simulink model "vehicle_hostmodel_2022b_RoadrunnerFinal"  (R2022b)
settings: Solver=VariableStepAuto  StartTime=0.0  StopTime=inf  RelTol=1e-3
model workspace (MAT data in the model file):
  finalint = 0
  firstWarning = 1
  originalScenarioChecksum = '114339432DE22364D47BB28FC96DC10C'
undefined symbols (not defined in the file): Acceleration, ActorID, AngularVelocity, curvature, DefaultGear, DEND_B, DEND_S, DEND_T, direction, DiscIntNeverNeededParam, driving, gradbp, L, LF, LR, matlabshared, MAX_BRAKE, MAX_STEER, MAX_TORQUE, MCAR, MIN_BRAKE, MIN_STEER, MIN_TORQUE, NUMD_B, NUMD_S, NUMD_T, Pitch, Position, psi_o, R, Roll, RRdamp, SceneInfo, session, sigbuilder_block, STEER_RATIO, stopSign_ID, Tdead, thetaRefs, TL_ID, TrackWidth, Ts, ts, Vdead, Velocity, WB, X_o, xRef2s, Y_o, Yaw, yRef2, yRef2s
libraries: simulink x10, drivingscenarioandsensors x8, slrealtimeutilitieslib x7, slrealtimeiplib x7, simulink_extras x4, drivingvehiclecontroller x3, robotalgslib x2, slpidlib x2, trackingutilitieslib x2, eeGeneralControl x1, mpcadaslib x1, drivinglib x1
(part 4 of 4)

== matlab function vehicle_hostmodel_2022b_RoadrunnerFinal/Function-Call Subsystem/MATLAB Function2 ==
  data: EgoPosition input; MIOPos input; curvature input; MIOVel input; V_i input; xd output; yd output; laneL input; laneR input; V_desired input; LCinProgress output
function [xd,yd,LCinProgress] = traj(EgoPosition,MIOPos,curvature,MIOVel, V_i, laneL, laneR, V_desired)
Vx_i =0;Vx_f=0;Vy_i=0;Vy_f=0;Ax_i=0;Ax_f=0;Ay_i=0;Ay_f=0;T_i=0;T_f=0;V_f=0;A_f=0;x_set=0;y_set=0;theta4=0;

P = zeros(6,6);
% xq = zeros(1,size(RefPath,1)); yq = zeros(1,size(RefPath,2));
EgoPosition(1,2)=-EgoPosition(1,2)
x_init= EgoPosition(1,1)+5; y_init = EgoPosition(1,2);
% xq = RefPath(:,1)'; 
% yq = RefPath(:,2)';
num_foc_t = 98;
V_max= V_desired; ad_n=0; vd_n=MIOVel; wd_n=vd_n*curvature;
lane_width = 3.6 * (laneL-laneR); % +1 if left of current lane and -1 if right of current lane
xd = zeros(num_foc_t+1,1); 
yd = zeros(num_foc_t+1,1);
xf =0; 
yf = 0;

    %xf = [EgoPosition(1,1)+ MIOPos(1) ]; yf = [ EgoPosition(1,2)+ MIOPos(2) + lane_width];  
    xf = [EgoPosition(1,1)+ 40 ]; yf = [ EgoPosition(1,2)+ 1.2*lane_width]; % 80
    V_f = V_max;
    W_f = V_f*curvature;
    A_f = 0;

    %dist2crash = sqrt((x_init-MIOPos(1))^2+(y_init-MIOPos(2))^2);
    %dist2crash = 40;
    %T_f = abs(dist2crash/(MIOVel-V_i));
    T_f = 3;
    P = [1, T_i, T_i^2, T_i^3, T_i^4, T_i^5;
         0, 1, 2*T_i, 3*T_i^2, 4*T_i^3, 5*T_i^4;
         0, 0, 2, 6*T_i, 12*T_i^2, 20*T_i^3;
         1, T_f, T_f^2, T_f^3, T_f^4, T_f^5;
         0, 1, 2*T_f, 3*T_f^2, 4*T_f^3, 5*T_f^4;
         0, 0, 2, 6*T_f, 12*T_f^2, 20*T_f^3];

%     mtang4 = (yq(1,index+2)-yq(1,index+1))/(xq(1,index+2)-xq(1,index+1));

    Vx_i = vd_n*cos(theta4); 
    Vy_i = vd_n*sin(theta4); 
    Ax_i = ad_n*cos(theta4)-vd_n*sin(theta4)*wd_n; 
    Ay_i = ad_n*sin(theta4)+vd_n*cos(theta4)*wd_n;

%     if(xq(index+2)-xq(index+1)<0)
%         theta_4 = pi + atan(mtang4);
%     else
%         theta_4 = atan(mtang4);
%     end

    theta_4 =0;
    Vx_f = V_f*cos(theta_4); % curvature angle
    Vy_f = V_f*sin(theta_4);
    Ax_f = A_f*cos(theta_4)-V_f*sin(theta_4)*W_f;
    Ay_f = A_f*sin(theta_4)+V_f*cos(theta_4)*W_f;

    g1 = [x_init; Vx_i; Ax_i; xf; Vx_f; Ax_f];
    g2 = [y_init; Vy_i; Ay_i; yf; Vy_f; Ay_f];

    a_coeff = P\g1;
    b_coeff = P\g2;
    
    td = T_i;
    scatter(x_init,y_init,'go')
    hold on; 
    scatter(xf,yf,'ro')
    hold on;
    
    for f = 1:(num_foc_t+1)
        xd(f,1) = [1,td,td^2,td^3,td^4,td^5]*a_coeff 
        yd(f,1) = [1,td,td^2,td^3,td^4,td^5]*b_coeff
        td = td + (T_f - T_i)/num_foc_t;
        scatter(xd(f,1),yd(f,1),'y.');
    end

LCinProgress = 1;

% hold on;
end

== matlab function vehicle_hostmodel_2022b_RoadrunnerFinal/Controllers/Subsystem3/Subsystem2/MATLAB Function ==
  data: u input; accel output; decel output
function [accel, decel] = fcn(u)
if(u>0)
    accel=u; decel=0;
elseif(u<0)
    accel=0; decel=-u;
else
    accel=0;decel=0;
end

== matlab function vehicle_hostmodel_2022b_RoadrunnerFinal/Controllers/MATLAB Function2 ==
  data: v input; RefVelCmd output; curvature input
function RefVelCmd = fcn(v,curvature)

    if abs(curvature) >= 0 && abs(curvature) <= 1e-2
        RefVelCmd = v;
    else
        r = 1/abs(curvature);
        RefVelCmd = min(v,sqrt(9.81*r*.2));
    end

== matlab function vehicle_hostmodel_2022b_RoadrunnerFinal/Vehicle Dynamics/Info2ActorState/MATLAB Function1 ==
  data: Xdot input; Velocity output; Ydot input; Zdot input
function Velocity = fcn(Xdot, Ydot, Zdot)

Velocity = [Xdot Ydot, Zdot];

== matlab function vehicle_hostmodel_2022b_RoadrunnerFinal/MATLAB Function ==
  data: ttc output; dist output; left output; right output; LL_avail output; RL_avail output; tend2stay output; ego input; act input; LaneBounds input; RoadSpeed input; ego_vel output; stay output; LL_Change output; RL_Change output; y_lane output; LCinProgress input
 function [ttc,dist,left,right,LL_avail,RL_avail,tend2stay,ego_vel,stay,LL_Change,RL_Change,y_lane] = fcn(ego,act,LaneBounds,RoadSpeed, LCinProgress)                       


%% Major tasks to look into

% Check the performance while transitioning into another lane 
% Lane change output when the ego on extreme lanes.
% Develop code to handle lane changes on road curvatures
% Integrate with the trajectory generation and check the perfomance 
% Convert the code to ego vehicle coordinates


%%
%define some parameters
r_c = 20; %range considered to MIOs
t_min =  2;

num_actors = length(act.Actors);
%num_lanes = length(LaneBounds.LaneBoundaries)-1;


%% Using sensor data 
% TracksNum = Tracking.NumTracks;
% 
% 
% for t = 1:TracksNum
%     ObjectID(t) = Tracking.Tracks(t).ObjectClassID;
%     TrackPos(:,t) = Tracking.Tracks(t).State(1:2:5);
%     TrackVel(:,t) = Tracking.Tracks(t).State(2:2:6);

%% ego position and  velocity magnitude
ego_pos = ego.Position;
ego_vel = ego.Velocity(1);  % velocity

%ttc: (array) : agent.relative position / abs(relative velocity)
ttc = zeros(1,num_actors);
left = zeros(1,num_actors);
right = zeros(1,num_actors);

dist =  zeros(1,num_actors);
tend2stay=1;

%%
y_lane = zeros(1,length(LaneBounds.LaneBoundaries))

for l=1:length(y_lane)
    y_lane(l)=LaneBounds.LaneBoundaries(l).Coordinates(end,2)
end

%%
for i= 1:num_actors

    % Grab actor positions and velocities
    actor_pos = act.Actors(i).Position;   
    actor_vel = act.Actors(i).Velocity(1);  % x-component velocity

    %relative velocity of the agent
    rel_vel = actor_vel - ego_vel;


    %% Check if the actor is within a r_c range. If it is out of range, pass lane change as '1' automatically.

   dist(i) = norm([actor_pos(1) actor_pos(2)]-[ego_pos(1) ego_pos(2)]);
        
    if dist(i) > r_c
        left(i)=1;
        right(i)=1;
        continue
    end

    %% Check if the actor is in the same lane as that of ego

    % If the actor and ego are in the same lane, it is considered a lead/following vehicle in the same lane and by defualt, the lane change flag is 1.

    if (actor_pos(2)< (ego_pos(2)+0.5) && actor_pos(2) > (ego_pos(2)-0.5))
        if (rel_vel < 0 && ego_vel < (RoadSpeed+5) && actor_pos(1) > ego_pos(1) )
            left(i) =1;
            right(i)=1;
            tend2stay=0;        % we need to incorporate too slow condition even when the relative velocity is greater than 0.

        elseif (rel_vel < 0 && ego_vel < (RoadSpeed+5) && actor_pos(1) < ego_pos(1) )
            left(i) =1;
            right(i)=1;
            tend2stay=1;
        end

        continue
    end

    
    %% calculate ttc for the rest of the vehicles


    ttc(i) = (actor_pos(1)-ego_pos(1))/abs(rel_vel);

    % checking conditions for other surrounding actors

    % all actors on the left lane of the ego vehicle
%%
    if actor_pos(2)-ego_pos(2) > 0  

        if and(rel_vel>0, ttc(i) > t_min)  % target vehicles on the front of ego vehicle (any lane)
    
            left(i)=1; 
            right(i)=1;
    
        elseif (ttc(i)<0 && rel_vel<0 && abs(ttc(i)) > t_min)    % target vehicle on the back of ego vehicle (ttc<0) (any lane)
            left(i) =1;
            right(i)=1;
    
        else 
            left(i) =0;
            right(i)=1;
    
        end

    % all actors on the right lane of the ego vehicle

    elseif actor_pos(2)-ego_pos(2) < 0
         
        if and(rel_vel>0, ttc(i) > t_min)  % target vehicles on the front of ego vehicle (any lane)
    
            left(i)=1;
            right(i)=1;
    
        elseif (ttc(i)<0 && rel_vel<0 && abs(ttc(i)) > t_min)    % target vehicle on the back of ego vehicle (ttc<0) (any lane)
            left(i) =1;
            right(i)=1;
    
        else 
            left(i) =1;
            right(i)=0;
    
        end
    end
%%

end

%% check if the vehicle is in the extreme end lanes

    if ego_pos(2)<y_lane(1) && ego_pos(2)>y_lane(2)

        LL=0; RL=1;
    elseif ego_pos(2) > y_lane(end) && ego_pos(2) < y_lane(end-1)
        RL=0; LL=1;
    else 

        RL=1;LL=1;
    end

%%
LL_avail = all(left) %&& LL;

RL_avail = all(right) %&& RL               %&& ~lcLeft ; this can be decided later 


%% final commands

stay = tend2stay || ~(tend2stay || LL_avail || RL_avail);
LL_Change =  ~tend2stay && LL_avail ;

RL_Change =  ~tend2stay && RL_avail && ~LL_Change ;
LCFlag = ~stay;
if LCFlag && LCinProgress
    LCFlag = false;
    stay = ~LCFlag;
end

%% 






end

== matlab function vehicle_hostmodel_2022b_RoadrunnerFinal/Vehicle Dynamics/Info2ActorState/MATLAB Function2 ==
  data: aX input; Acceleration output; aY input; aZ input
function Acceleration = fcn(aX, aY, aZ)

Acceleration = [aX aY, aZ];

== matlab function vehicle_hostmodel_2022b_RoadrunnerFinal/Vehicle Dynamics/Info2ActorState/MATLAB Function3 ==
  data: phiDot input; AngularVelocity output; thetaDot input; psiDot input
function AngularVelocity = fcn(phiDot, thetaDot, psiDot)

AngularVelocity = [phiDot thetaDot, psiDot];

== stateflow chart vehicle_hostmodel_2022b_RoadrunnerFinal/Vehicle Dynamics/VehicleDynamics/engine-steer-brake dynamics/GearSelection1 ==
  state Park
    CurrGear = 0;
  state Reverse
    CurrGear = -1;
  state drive
    CurrGear = 1;
  (default) -> (junction 12)
  (junction 12) -> Reverse [order 3] : [DefaultGear == -1]
  (junction 12) -> drive [order 2] : [DefaultGear == 1]
  (junction 12) -> Park [order 1] : [DefaultGear == 0]
  (junction 12) -> Park [order 4] : %fallback to park
  drive -> Park [order 2] : [gear_cmd == 0 && allowShift(vc,Tbrake)]
  Park -> Reverse [order 2] : [gear_cmd == -1 && allowShift(vc,Tbrake)]
  Park -> drive [order 1] : [gear_cmd == 1 && allowShift(vc,Tbrake)]
  Reverse -> Park [order 2] : [gear_cmd == 0 && allowShift(vc,Tbrake)]
  drive -> Reverse [order 1] : [gear_cmd == -1 && allowShift(vc,Tbrake)]
  Reverse -> drive [order 1] : [gear_cmd == 1 && allowShift(vc,Tbrake)]
  data: Tdead parameter; Vdead parameter; vel function_input; brakeT function_input; allow function_output; CurrGear output; Tbrake input; vc input; gear_cmd input; DefaultGear parameter
  function allow = allowShift(vel, brakeT):
    | function allow = allowShift(vel, brakeT)
    | allow = (abs(vel) <= Vdead) && (abs(brakeT)>Tdead);
    | end

== matlab function vehicle_hostmodel_2022b_RoadrunnerFinal/Vehicle Dynamics/VehicleDynamics/engine-steer-brake dynamics/compute net torque ==
  data: gear input; Tnet output; Tengine input; Tbrake input; vc input
function Tnet  = net_torque(gear,Tengine,Tbrake,vc)

%  --set engine torque based on current gear selection

if (gear == 0)
    %  --vehicle is in PARK, so force engine torque to zero
    Tengine = 0;
end

Tnet = Tengine + Tbrake*tanh(5*vc);

end

== matlab function vehicle_hostmodel_2022b_RoadrunnerFinal/Vehicle Dynamics/VehicleDynamics/engine-steer-brake dynamics/gear selection state machine ==
  data: gear output; gear_cmd input; vc input; Tbrake input; Tdead input; Vdead input
function gear = gear_change_FSM(gear_cmd,vc,Tbrake,Tdead,Vdead)

persistent GEAR

%  The vehicle gear can take on one of the following enumerated values:
%  -1 = REVERSE
%   0 = PARK
%   1 = DRIVE

%  --initialize the local persistent variables

if isempty(GEAR)
    %  --default gear at startup is PARK
    %  Note:  Change this to 1 if you want car to initialize in DRIVE
    GEAR = 0;
end


%  --evaluate the gear change finite state machine

switch GEAR
    case 0  % vehicle is in PARK
        if (gear_cmd == 1)
            %  --check to see if we can shift to DRIVE
            if ((abs(vc) <= Vdead) && (abs(Tbrake) > Tdead))
                %  --shift to DRIVE
                GEAR = 1;
            end
            
        elseif (gear_cmd == 2)
            %  --check to see if we can shift to REVERSE
            if ((abs(vc) <= Vdead) && (abs(Tbrake) > Tdead))
                %  --shift to REVERSE
                GEAR = 2;
            end
        end
        
    case 1  % vehicle is in DRIVE
        if (gear_cmd == 0)
            %  --check to see if we can shift to PARK
            if ((abs(vc) <= Vdead) && (abs(Tbrake) > Tdead))
                %  --shift to PARK
                GEAR = 0;
            end
            
        elseif (gear_cmd == 2)
            %  --check to see if we can shift to REVERSE
            if ((abs(vc) <= Vdead) && (abs(Tbrake) > Tdead))
                %  --shift to REVERSE
                GEAR = 2;
            end
        end
        
    case -1  % vehicle is in REVERSE
        if (gear_cmd == 0)
            %  --check to see if we can shift to PARK
            if ((abs(vc) <= Vdead) && (abs(Tbrake) > Tdead))
                %  --shift to PARK
                GEAR = 0;
            end
            
        elseif (gear_cmd == 1)
            %  --check to see if we can shift to DRIVE
            if ((abs(vc) <= Vdead) && (abs(Tbrake) > Tdead))
                %  --shift to DRIVE
                GEAR = 1;
            end
        end
        
    otherwise  %  --should never be here
        if (vc > Vdead)
            %  --moving forward, so must be in DRIVE
            GEAR = 1;
        elseif (vc < -Vdead)
            %  --moving backward, so must be in REVERSE
            GEAR = 2;
        else
            %  --vehicle stoppped, so must be in PARK
            GEAR = 0;
        end

end


%  --output the current actual gear setting

gear = GEAR;

return

== matlab function vehicle_hostmodel_2022b_RoadrunnerFinal/Controllers/Lateral Controllers1/Swicth 1 ==
  data: stan input; y output; pure input
function y = fcn(stan, pure)

if stan<pure
    y=stan
else
    y=pure
end

== matlab function vehicle_hostmodel_2022b_RoadrunnerFinal/Controllers/Lateral Controllers1/Average ==
  data: stan input; y output; pure input
function y = fcn(stan, pure)

y=(stan+pure)/2

== matlab function vehicle_hostmodel_2022b_RoadrunnerFinal/Function-Call Subsystem/MATLAB Function1 ==
  data: EgoPosition input; MIOPos input; curvature input; MIOVel input; V_i input; xd output; yd output; laneL input; laneR input; V_desired input; LCinProgress output
function [xd,yd,LCinProgress] = traj(EgoPosition,MIOPos,curvature,MIOVel, V_i, laneL, laneR, V_desired)
Vx_i =0;Vx_f=0;Vy_i=0;Vy_f=0;Ax_i=0;Ax_f=0;Ay_i=0;Ay_f=0;T_i=0;T_f=0;V_f=0;A_f=0;x_set=0;y_set=0;theta4=0;

P = zeros(6,6);
% xq = zeros(1,size(RefPath,1)); yq = zeros(1,size(RefPath,2));
EgoPosition(1,2)=-EgoPosition(1,2);
x_init= EgoPosition(1,1)+2; y_init = EgoPosition(1,2)-2;
% xq = RefPath(:,1)'; 
% yq = RefPath(:,2)';
num_foc_t = 98;
V_max= V_desired; ad_n=0; vd_n=MIOVel; wd_n=vd_n*curvature;
lane_width = 3.6 * (laneL-laneR); % +1 if left of current lane and -1 if right of current lane(rahul flipped)
xd = zeros(num_foc_t+1,1); 
yd = zeros(num_foc_t+1,1);
xf =0; 
yf = 0;

    %xf = [EgoPosition(1,1)+ MIOPos(1) ]; yf = [ EgoPosition(1,2)+ MIOPos(2) + lane_width];  
    xf = [EgoPosition(1,1)+ 20 ]; yf = [EgoPosition(1,2)+ lane_width]; % 80
    V_f = V_max;
    W_f = V_f*curvature;
    A_f = 0;

    %dist2crash = sqrt((x_init-MIOPos(1))^2+(y_init-MIOPos(2))^2);
    %dist2crash = 40;
    %T_f = abs(dist2crash/(MIOVel-V_i));
    T_f = 3;
    P = [1, T_i, T_i^2, T_i^3, T_i^4, T_i^5;
         0, 1, 2*T_i, 3*T_i^2, 4*T_i^3, 5*T_i^4;
         0, 0, 2, 6*T_i, 12*T_i^2, 20*T_i^3;
         1, T_f, T_f^2, T_f^3, T_f^4, T_f^5;
         0, 1, 2*T_f, 3*T_f^2, 4*T_f^3, 5*T_f^4;
         0, 0, 2, 6*T_f, 12*T_f^2, 20*T_f^3];

%     mtang4 = (yq(1,index+2)-yq(1,index+1))/(xq(1,index+2)-xq(1,index+1));

    Vx_i = vd_n*cos(theta4); 
    Vy_i = vd_n*sin(theta4); 
    Ax_i = ad_n*cos(theta4)-vd_n*sin(theta4)*wd_n; 
    Ay_i = ad_n*sin(theta4)+vd_n*cos(theta4)*wd_n;

%     if(xq(index+2)-xq(index+1)<0)
%         theta_4 = pi + atan(mtang4);
%     else
%         theta_4 = atan(mtang4);
%     end

    theta_4 =0;
    Vx_f = V_f*cos(theta_4); % curvature angle
    Vy_f = V_f*sin(theta_4);
    Ax_f = A_f*cos(theta_4)-V_f*sin(theta_4)*W_f;
    Ay_f = A_f*sin(theta_4)+V_f*cos(theta_4)*W_f;

    g1 = [x_init; Vx_i; Ax_i; xf; Vx_f; Ax_f];
    g2 = [y_init; Vy_i; Ay_i; yf; Vy_f; Ay_f];

    a_coeff = P\g1;
    b_coeff = P\g2;
    
    td = T_i;
    scatter(x_init,y_init,'go')
    hold on; 
    scatter(xf,yf,'ro')
    hold on;
    
    for f = 1:(num_foc_t+1)
        xd(f,1) = [1,td,td^2,td^3,td^4,td^5]*a_coeff 
        yd(f,1) = [1,td,td^2,td^3,td^4,td^5]*b_coeff
        td = td + (T_f - T_i)/num_foc_t;
        scatter(xd(f,1),yd(f,1),'y.');
    end

LCinProgress = 1;

% hold on;
end

== matlab function vehicle_hostmodel_2022b_RoadrunnerFinal/Turns LC in prog off ==
  data: u input; y output
function y = fcn(u)

persistent counter;
persistent input_high;

if isempty(counter)
    counter = 0;
end

if isempty(input_high)
    input_high = false;
end

if u ~= 0
    input_high = true;
end

if input_high && counter < 100
    y = u;
    counter = counter + 1;
else
    y = 0;
end

== matlab function vehicle_hostmodel_2022b_RoadrunnerFinal/Controllers/Lateral Controllers/Subsystem1/MATLAB Function3 ==
  data: velocity input; L_tune output; L_min input; L_max input; velocity_gain input; error_gain input; lateral_error input
function L_tune = fcn(velocity,L_min,L_max,velocity_gain,error_gain,lateral_error)

    if velocity<=5
        L_tune = L_min;
    elseif velocity >5 && velocity<15
        L_chk = abs(velocity_gain*abs(velocity)-error_gain*lateral_error);
        if L_chk < L_min
            L_tune = L_min
        else
            L_tune = L_chk
        end
    else
        L_tune = abs(L_max-error_gain*lateral_error);
    end

== matlab function vehicle_hostmodel_2022b_RoadrunnerFinal/Controllers/Lateral Controllers/Subsystem1/MATLAB Function4 ==
  settings: updateMethod=DISCRETE
  data: K_out output; current_ref output; r output; theta_p output; cross_track_error output; old_index output; current_error_chk output; lookahead_distance input; pose input; waypoints input; D_sat input; old_index input; new_wp output
function [K_out,current_ref,r,theta_p,cross_track_error,old_index,current_error_chk,new_wp] = fcn(lookahead_distance,pose,waypoints,D_sat,old_index)
    min_ = inf;
    current_ref = zeros(1,2);

    idx = 0;
    id = old_index;

    for j=1:length(waypoints)
        if norm(pose(1:2)-waypoints(j,1:2))<min_
           min_ = norm(pose(1:2)-waypoints(j,1:2));
           current_ref = waypoints(j,1:2);
           idx = j;
           end
    end
    
    old_index = idx;

    new_wp = zeros(1,2);

    flagk = 0;

    for k=idx:length(waypoints)
        if norm(current_ref-waypoints(k,1:2)) > lookahead_distance
            new_wp = waypoints(k,:);
            flagk = 1;
            break  
        end
    end

    if flagk == 0
        min_l = inf;
        new_index = 0
        for l = length(waypoints):-1:(idx+1)
            if norm(current_ref-waypoints(l,1:2))<=min_l
                min_l = norm(current_ref-waypoints(l,1:2));
                new_index = l;
            end
        end
        new_wp = waypoints(l,1:2);
    end 
    
    theta_p = atan2d((new_wp(1,2)-current_ref(1,2)),(new_wp(1,1)-current_ref(1,1)));

    current_heading = pose(1,3);

    lookahead_angle = (theta_p-current_heading);

    d_new = 0;
    d_calc = 0;

    A = [cosd(theta_p+pi/2) -cosd(current_heading+lookahead_angle);sind(theta_p+pi/2) -sind(current_heading+lookahead_angle)];

    vec_dif = current_ref-new_wp;

    new_vec = zeros(2,1);

    if det(A)>1e-5
        new_vec = A\vec_dif';
        d_calc = new_vec(1,1);
        if d_calc>=D_sat
            d_new = sign(d_calc)*D_sat;
        else
            d_new = d_calc;
        end

        wp_sel = new_wp - [d_new*cosd(theta_p+pi/2) d_new*sind(theta_p+pi/2)];
    else
        wp_sel = new_wp;
    end

    vec_car_frame = [cosd(current_heading) sind(current_heading);-sind(current_heading) cosd(current_heading)]*(wp_sel'-current_ref');

    r = lookahead_distance^2/(2*vec_car_frame(2,1));

    K_out = 1/r;

  
    %{
    if abs(old_curvature) < 0.01 & abs(K_computed) < 0.01
        K_out = 0;
    else
        K_out = K_computed;
    end
    %}
    
   


    K_ref = 2*sind(lookahead_angle)/lookahead_distance;
    

    
    cross_track_error = vec_car_frame(2,1);

    computed_error =  norm(current_ref'-pose(1:2)');

  
    if computed_error<0.01
        current_error_chk = 0;
    else
        current_error_chk = computed_error;
    end

== matlab function vehicle_hostmodel_2022b_RoadrunnerFinal/Controllers/Lateral Controllers/Subsystem1/MATLAB Function5 ==
  data: error_la output; Lad input; theta_p input; pose input; cross_track_error input; L input
function error_la = fcn(Lad,theta_p,pose,cross_track_error,L)
    current_angle = pose(3);
    heading_error = theta_p-current_angle;
    error_la = cross_track_error+(L/2+Lad)*sind(heading_error);

== matlab function vehicle_hostmodel_2022b_RoadrunnerFinal/Controllers/Lateral Controllers/Subsystem1/MATLAB Function6 ==
  data: r input; theta output; L input
function theta = fcn(r,L)

theta = atan(L/r);

== matlab function vehicle_hostmodel_2022b_RoadrunnerFinal/PathPlanner/MATLAB Function3 ==
  settings: updateMethod=DISCRETE
  data: out output; check output; Xref input; Yref input; xd input; yd input; LC input; current_pos input; d2f input; dcheck output
function [out,check,dcheck]  = PathPlanning(Xref, Yref, xd, yd, LC, current_pos, d2f)

persistent output_matrix
persistent lc_triggered

if isempty(lc_triggered)
lc_triggered = false;
end

%lc_triggered=0;
%if isempty(hold_output)
  %  hold_output = false;
%end


if isempty(output_matrix)
    output_matrix = [Xref(:), Yref(:)];
    out = [Xref(:), Yref(:)];
else
    out = output_matrix;
end

if LC && ~isempty(xd) && ~isempty(yd)
    output_matrix = [xd(:), yd(:)];
    lc_triggered=true;
       
end

check=lc_triggered;
dcheck=output_matrix;
%out=output_matrix;

if lc_triggered && d2f < 5 %&& ~isempty(output_matrix) %&& ~hold_output
    %Yout = Yref(:);
    if current_pos > 0
        Xout = Xref(:);
        Yout = Yref + 3.6;
    else
        Xout = Xref(:);
        Yout = Yref;
    end
    output_matrix = [Xout, Yout];
    out=output_matrix;
    lc_triggered=false;
    %hold_output = true;
end

out=output_matrix;




%if ~LC && ~isempty(output_matrix) && lc_triggered
    %hold_output = false;
    %lc_triggered=false;
%end

end

== stateflow chart vehicle_hostmodel_2022b_RoadrunnerFinal/Behavioural Planner2/Chart ==
  settings: updateMethod=DISCRETE  sampleTime=Ts
  state Stationary
    du:
    VelCmd = 0;
    CurrentVelCmd = VelCmd;
    Navi = 0;
    Trans = 0;
    StopSim = 0;
  state Navigation
    state RailCrossing
      state Approaching
        en:
        ACC = 1;
        Tgap = 0;
        Trans = 0;
      state Stop
        en:
        VelCmd = 0;
        ACC = 0;
        CurrentVelCmd = VelCmd;
      state ExitScene
        en:
        ExitFlag = 1;
      state Transition
        en:
        Tgap = 1;
        Trans = 1;
        VelCmd = SceneSpeed;
        CurrentVelCmd = VelCmd;
      (default) -> Navigation.RailCrossing.Approaching
      Navigation.RailCrossing.Approaching -> Navigation.RailCrossing.Stop [order 1] : [D2S <= 4]
      Navigation.RailCrossing.Stop -> Navigation.RailCrossing.Transition : [RRCross == 0]
      Navigation.RailCrossing.Approaching -> Navigation.RailCrossing.ExitScene [order 2] : [SceneID ~= 10]
      Navigation.RailCrossing.Transition -> Navigation.RailCrossing.ExitScene : [SceneID == 0]
    state RoundAbout
      state Approaching
        en:
        ACC = 1;
        Trans = 0;
        Tgap = 0;
      state Stop
        en:
        VelCmd = 0;
        ACC = 0;
        CurrentVelCmd = VelCmd;
      state ExitScene
        en:
        ExitFlag = 1;
      state Transition
        en:
        Tgap = 1;
        Trans = 1;
        VelCmd = SceneSpeed;
        CurrentVelCmd = VelCmd;
      (default) -> Navigation.RoundAbout.Approaching
      Navigation.RoundAbout.Approaching -> Navigation.RoundAbout.Stop [order 1] : [D2S <= 4]
      Navigation.RoundAbout.Stop -> Navigation.RoundAbout.Transition : [Clear2Go == 1]
      Navigation.RoundAbout.Approaching -> Navigation.RoundAbout.ExitScene [order 2] : [SceneID ~= 9]
      Navigation.RoundAbout.Transition -> Navigation.RoundAbout.ExitScene : [SceneID == 0]
    state DestCheck
      en,du:
      % dest reached?
      (default) -> (junction 47)
      (junction 47) -> (junction 48) [order 1] : [D2D < 2]
      (junction 48) -> (junction 50) : {DestReached = 1;}
      (junction 47) -> (junction 49) [order 2] : {DestReached = 0;}
      (junction 50) -> (junction 49) : {StopSim = 1;}
      (junction 49) -> (junction 51)
    state TrafficLight
      state Stop
        en:
        %CurrentVelCmd = VelCmd;
        %du:
        %if D2S < 7
        % VelCmd = 0;
        %end
      state Approaching
        en:
        Tgap = 0;
        Trans = 0;
        %if TLstate(1,4) == 1
        ACC = 1;
        %else
        % ACC = 0;
        %end
      state Transition
        en:
        Trans = 1;
        ACC = 0;
        Tgap = 1;
        VelCmd = SceneSpeed;
        CurrentVelCmd = VelCmd;
      state ExitScene
        en:
        ExitFlag = 1;
      (default) -> Navigation.TrafficLight.Approaching
      Navigation.TrafficLight.Approaching -> Navigation.TrafficLight.Stop [order 1] : [D2S <= 4]
      Navigation.TrafficLight.Transition -> Navigation.TrafficLight.Approaching [order 2] : [TLstate(1,4) == 1]
      Navigation.TrafficLight.Stop -> Navigation.TrafficLight.Transition : [TLstate(1,4) == 3]
      Navigation.TrafficLight.Approaching -> Navigation.TrafficLight.Transition [order 2] : [TLstate(1,4) == 3]
      Navigation.TrafficLight.Approaching -> Navigation.TrafficLight.ExitScene [order 3] : [SceneID ~= 8]
      Navigation.TrafficLight.Transition -> Navigation.TrafficLight.ExitScene [order 1] : [SceneID == 0]
    state SceneRecognition
      en :
      VelCmd = RoadSpeed;
      CurrentVelCmd = VelCmd;
      ExitFlag = 0;
    state Go
      en:
      VelCmd = RoadSpeed;
      CurrentVelCmd = VelCmd;
      Trans = 0;
      ExitFlag = 0;
      ACC = 0;
    state StopSign
      state Approaching
        en:
        ACC = 1;
        Trans = 0;
        Tgap = 0;
      state Stop
        en:
        VelCmd = 0;
        ACC = 0;
        CurrentVelCmd = VelCmd;
      state ExitScene
        en:
        ExitFlag = 1;
      state Transition
        en:
        Trans = 1;
        ACC = 0;
        Tgap = 1;
        VelCmd = SceneSpeed;
        CurrentVelCmd = VelCmd;
      (default) -> Navigation.StopSign.Approaching
      Navigation.StopSign.Approaching -> Navigation.StopSign.Stop [order 1] : [D2S <= 7]
      Navigation.StopSign.Stop -> Navigation.StopSign.Transition : [after(3,sec) && Clear2Go == 1]
      Navigation.StopSign.Approaching -> Navigation.StopSign.ExitScene [order 2] : [SceneID ~= 7]
      Navigation.StopSign.Transition -> Navigation.StopSign.ExitScene : [SceneID == 0]
    Go -> RailCrossing [order 2] : [SceneID == 10]
    SceneRecognition -> RailCrossing [order 1] : [SceneID == 10]
    RailCrossing -> Go : [ExitFlag == 1]
    Go -> RoundAbout [order 4] : [SceneID == 9]
    SceneRecognition -> RoundAbout [order 2] : [SceneID == 9]
    RoundAbout -> Go : [ExitFlag == 1]
    (default) -> DestCheck
    SceneRecognition -> TrafficLight [order 4] : [SceneID == 8]
    DestCheck -> SceneRecognition : [DestReached == 0]
    Go -> TrafficLight [order 3] : [SceneID == 8]
    SceneRecognition -> DestCheck [order 5] : [D2D < 2]
    SceneRecognition -> StopSign [order 3] : [SceneID == 7]
    TrafficLight -> Go : [ExitFlag == 1]
    StopSign -> Go : [ExitFlag == 1]
    Go -> DestCheck [order 1] : [SceneID == 0]
    Go -> StopSign [order 5] : [SceneID == 7]
  (default) -> Stationary
  Stationary -> Navigation : [Navigate == 1]
  Navigation -> Stationary : [Navigate == 0 || DestReached == 1]
  data: TLstate input; ApproachingSpeed input; ObjectDist input; SceneSpeed input; SDist input; RRCross input; D2S input; DestReached local; Navigate input; ExitFlag local; D2D input; Clear2Go input; RoadSpeed input; CurrentVelCmd local; Navi local; VelCmd output; SceneID input; ACC output; Tgap output; Trans output; StopSim output

== stateflow chart vehicle_hostmodel_2022b_RoadrunnerFinal/Behavioural Planner2/Collision Avoidance ==
  state Start
    en:
    Stuck = 0;
    ACC = 0;
    LaneChangeCmd = 0;
    %VelCmd = CurrentVelCmd;
  state Follow
    en:
    ACC = 1;
  state LaneChange
    en:
    LaneChangeCmd = 1;
    ACC=0;
  LaneChange -> Start : [LaneChanged == 1]
  (default) -> Start
  Follow -> LaneChange [order 2] : [LaneAvailable == 1 && Stuck == 1]
  Start -> Follow : [ObjAhead == 1]
  Follow -> Start [order 3] : [ObjAhead == 0]
  Follow -> Follow [order 1] : [(EgoSpeed <= MinSpeed) && after(WaitTime,sec)]{Stuck = 1;}
  data: Stuck local; ACC output; WaitTime input; ObjAhead input; MinSpeed input; LaneAvailable input; EgoSpeed input; LaneChanged input; LaneChangeCmd output

== stateflow chart vehicle_hostmodel_2022b_RoadrunnerFinal/Behavioural Planner2/Emergency Stop ==
  state EmergencyCheck
    en:
    EStop = 0;
  state Pullover
    en:
    EStop=1;
  state Stop
    en:
    EStop=2;
  Pullover -> EmergencyCheck : [TechFailure == 0]
  (default) -> EmergencyCheck
  EmergencyCheck -> Pullover [order 1] : [TechFailure == 1]
  EmergencyCheck -> Stop [order 2] : [D2O<=1]
  Stop -> EmergencyCheck : [D2O > 2]
  data: D2O input; TechFailure input; EStop output

== matlab function vehicle_hostmodel_2022b_RoadrunnerFinal/Behavioural Planner2/MATLAB Function ==
  data: Dest input; D2D output; CurrentPose input
function D2D = fcn(Dest, CurrentPose)
CurrentPose(2) = CurrentPose(2);    %Change sign to negative if flipping signs in tlstart ref pose.
D2D = norm(Dest - CurrentPose(1:2)');

== stateflow chart vehicle_hostmodel_2022b_RoadrunnerFinal/Behavioural Planner2/Routing ==
  state InitialRoute
    en:
    NewRoute = 0;
  state Rerouting
    en:
    NewRoute = 1;
  (default) -> InitialRoute
  InitialRoute -> Rerouting : [ReRoute == 1]
  Rerouting -> InitialRoute : [ReRoute == 0]
  data: ReRoute input; NewRoute output
